simulink model "lab3"  (R2016a)
settings: Solver=FixedStepDiscrete  StartTime=0.0  StopTime=inf  FixedStep=0.025  RelTol=1e-3
PostLoadFcn:
  | init_lab3
InitFcn:
  | if IMU_Kalman_D.a==0
  |   IMU_Kalman_D.Ts = Ts;
  | end
  | if Wheel_Kalman_D.a==0
  |   Wheel_Kalman_D.Ts = Ts;
  | end
values from neighbouring files (symbols this model uses):
  Feedback_Gain = [0 0 0 0]    [init_lab3.m]
  Integral_Gain = 0    [init_lab3.m]
  Ts = 0.025    [init_lab3.m]
undefined symbols (not defined in the file or in its folder): DiscIntNeverNeededParam
libraries: cstblocks x2, MinSegLibrary_M1V4 x2, simulink x1
settings Model: SimulationMode=external  ExtModeTrigDuration=2  Creator=Alec  LastModifiedBy=nilsv
settings DataIOCC: LimitDataPoints=on  SaveFormat=Array  SaveOutput=off  SignalLogging=off  DSMLogging=off  VisualizeSimOutput=off  SaveTime=off
settings OptimizationCC: PassReuseOutputArgsThreshold=0  ExpressionDepthLimit=2147483647  MaxStackSize=64
settings DebuggingCC: UnderspecifiedInitializationDetection=Classic  MergeDetectMultiDrivingBlocksExec=none  ParameterTunabilityLossMsg=error  UnconnectedInputMsg=none  UnconnectedOutputMsg=none  StateNameClashWarn=warning
settings HardwareCC: ProdBitPerInt=16  ProdBitPerPointer=16  ProdLargestAtomicFloat=None  ProdWordSize=8  ProdHWDeviceType=Atmel->AVR  UseEmbeddedCoderFeatures=off  UseSimulinkCoderFeatures=off
settings ModelReferenceCC: PropagateSignalLabelsOutOfModel=off
settings RTWCC: SystemTargetFile=ert.tlc  HardwareBoard=Arduino Mega 2560  TLCOptions=-aInlineSetEventsForThisBaseRateFcn=TLC_FALSE -aSuppressMultiTaskScheduler=TLC_FALSE -aRateBasedStepFcn=1  TemplateMakefile=ert_default_tmf  GenerateReport=on  RTWVerbose=off  Toolchain=Arduino AVR v1.6.1  BuildConfiguration=Faster Runs  LaunchReport=on
settings CodeAppCC: ForceParamTrailComments=on  OperatorAnnotations=on  MangleLength=10
settings ERTTargetCC: MultiwordLength=256  ERTCustomFileBanners=off  SupportContinuousTime=on  SupportNonInlinedSFcns=on  SupportVariableSizeSignals=on  ModelStepFunctionPrototypeControlCompliant=off
settings ConfigComp: CovEnableCumulative=off  CovSaveSingleToWorkspaceVar=off  CovSaveOutputData=off

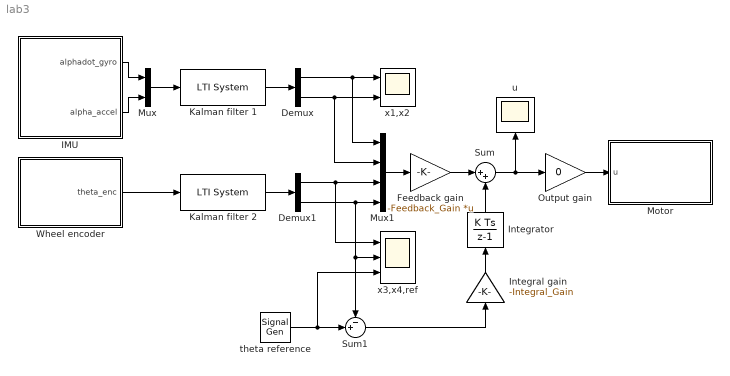
== system lab3 ==
  Demux : Demux  Outputs=2
  Demux1 : Demux  Outputs=2
  Feedback gain : Gain  Gain=-Feedback_Gain  Multiplication=Matrix(K*u)
  IMU : Subsystem
  Integral gain : Gain  Gain=-Integral_Gain
  Integrator : DiscreteIntegrator  gainval=1  InitialConditionSetting=State (most efficient)  SampleTime=-1  ICPrevOutput=DiscIntNeverNeededParam  ICPrevScaledInput=DiscIntNeverNeededParam
  Kalman filter 1 : cstblocks/LTI System  sys=IMU_Kalman_D  IC=[]
  Kalman filter 2 : cstblocks/LTI System  sys=Wheel_Kalman_D  IC=[]
  Motor : Subsystem
  Mux : Mux  Inputs=2
  Mux1 : Mux
  Output gain : Gain  Gain=0
  Sum : Sum  Inputs=|++
  Sum1 : Sum  Inputs=-+|
  Wheel encoder : Subsystem
  theta reference : SignalGenerator  WaveForm=square  Amplitude=0  Frequency=0.025
  u : Scope
  x1,x2 : Scope  NumInputPorts=2
  x3,x4,ref : Scope  NumInputPorts=3
  wires:
  Mux/1 -> Kalman filter 1/1
  Kalman filter 1/1 -> Demux/1
  Demux/2 -> Mux1/2, x1,x2/2
  Demux/1 -> Mux1/1, x1,x2/1
  Mux1/1 -> Feedback gain/1
  Wheel encoder/1(theta_enc) -> Kalman filter 2/1
  Demux1/1 -> Mux1/3, x3,x4,ref/1
  Demux1/2 -> Sum1/1, x3,x4,ref/2, Mux1/4
  Kalman filter 2/1 -> Demux1/1
  Output gain/1 -> Motor/1(u)
  Feedback gain/1 -> Sum/1
  Sum/1 -> u/1, Output gain/1
  theta reference/1 -> x3,x4,ref/3, Sum1/2
  IMU/2(alpha_accel) -> Mux/2
  IMU/1(alphadot_gyro) -> Mux/1
  Integrator/1 -> Sum/2
  Integral gain/1 -> Integrator/1
  Sum1/1 -> Integral gain/1

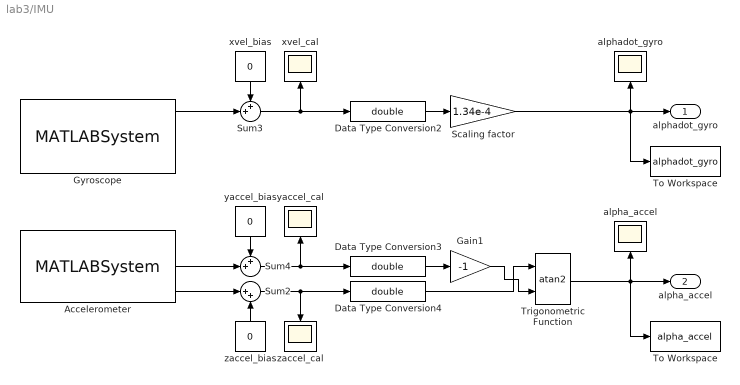
== system lab3/IMU ==
  " To Workspace " : ToWorkspace  VariableName=alpha_accel  SampleTime=-1
      settings: Save2DSignal=2-D array (concatenate along first dimension)
  Accelerometer : MATLABSystem  System=soMPU6050Accel  SimulateUsing=Code generation
      mask Type: soMPU6050Accel
      mask Display:
      | disp('soMPU6050Accel');
      | port_label('output',1,'xaccel');
      | port_label('output',2,'yaccel');
      | port_label('output',3,'zaccel');
  Data Type Conversion2 : DataTypeConversion  OutDataTypeStr=double
  Data Type Conversion3 : DataTypeConversion  OutDataTypeStr=double
  Data Type Conversion4 : DataTypeConversion  OutDataTypeStr=double
  Gain1 : Gain  Gain=-1
  Gyroscope : MATLABSystem  System=soMPU6050Gyro  DLPFmode=0
      mask Type: soMPU6050Gyro
      mask Display:
      | disp('soMPU6050Gyro');
      | port_label('output',1,'xvel');
      | port_label('output',2,'yvel');
      | port_label('output',3,'zvel');
  Scaling factor : Gain  Gain=1.34e-4
  Sum2 : Sum  Inputs=|++
  Sum3 : Sum  Inputs=++|
  Sum4 : Sum  Inputs=++|
  To Workspace : ToWorkspace  VariableName=alphadot_gyro  SampleTime=-1
      settings: Save2DSignal=2-D array (concatenate along first dimension)
  Trigonometric Function : Trigonometry  Operator=atan2
  "alpha_accel " : Scope
  "alphadot_gyro " : Scope
  xvel_bias : Constant  Value=0
  xvel_cal : Scope
  yaccel_bias : Constant  Value=0
  yaccel_cal : Scope
  zaccel_bias : Constant  Value=0
  zaccel_cal : Scope
  alphadot_gyro : Outport
  alpha_accel : Outport  Port=2
  wires:
  zaccel_bias/1 -> Sum2/2
  Gyroscope/1 -> Sum3/2
  Sum3/1 -> xvel_cal/1, Data Type Conversion2/1
  Data Type Conversion2/1 -> Scaling factor/1
  Scaling factor/1 -> "alphadot_gyro "/1, alphadot_gyro/1, To Workspace/1
  xvel_bias/1 -> Sum3/1
  Accelerometer/2 -> Sum4/2
  Sum4/1 -> yaccel_cal/1, Data Type Conversion3/1
  yaccel_bias/1 -> Sum4/1
  Accelerometer/3 -> Sum2/1
  Sum2/1 -> zaccel_cal/1, Data Type Conversion4/1
  Data Type Conversion3/1 -> Gain1/1
  Data Type Conversion4/1 -> Trigonometric Function/1
  Gain1/1 -> Trigonometric Function/2
  Trigonometric Function/1 -> " To Workspace "/1, alpha_accel/1, "alpha_accel "/1

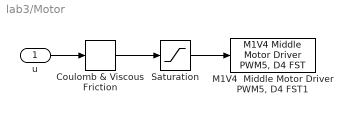
== system lab3/Motor ==
  u : Inport
  Coulomb & Viscous Friction : simulink/Discontinuities/Coulomb & Viscous Friction  offset=0.25  gain=1
  "M1V4  Middle Motor Driver PWM5, D4 FST1" : MinSegLibrary_M1V4/M1V4  Middle Motor Driver PWM5, D4 FST  Vsupply=3.25
  Saturation : Saturate  UpperLimit=3.25  LowerLimit=-3.25
  wires:
  u/1 -> Coulomb & Viscous Friction/1
  Coulomb & Viscous Friction/1 -> Saturation/1
  Saturation/1 -> "M1V4  Middle Motor Driver PWM5, D4 FST1"/1

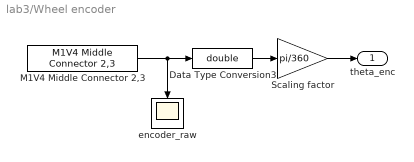
== system lab3/Wheel encoder ==
  Data Type Conversion3 : DataTypeConversion  OutDataTypeStr=double
  M1V4 Middle Connector 2,3 : MinSegLibrary_M1V4/M1V4 Middle Connector 2,3  Encoder=0  PinA=3  PinB=2
  Scaling factor : Gain  Gain=pi/360
  encoder_raw : Scope
  theta_enc : Outport
  wires:
  Data Type Conversion3/1 -> Scaling factor/1
  Scaling factor/1 -> theta_enc/1
  M1V4 Middle Connector 2,3/1 -> encoder_raw/1, Data Type Conversion3/1
